simulink model "Kinematic"  (R2023b)
settings: Solver=VariableStepAuto  StartTime=0.0  StopTime=10.0  RelTol=1e-3
values from neighbouring files (symbols this model uses):
  dQ1 = x(6)    [BSM.m]    (also in Correct_new_data.m; MechanicalMechanics_Dynamic.m; MechanicalMechanics_Dynamic_adaptive_BSM.m; MechanicalMechanics_Kinematics.m)
  L1 = x(1)    [Adams_HW1.m]    (also in Adams_HW_DrawGIF.m = current_x(1); Adams_HW_DrawGIF_Y.m = current_x(1); BSM.m; Correct_new_data.m)
  L2 = x(2)    [Adams_HW1.m]    (also in Adams_HW_DrawGIF.m = current_x(2); Adams_HW_DrawGIF_Y.m = current_x(2); BSM.m; Correct_new_data.m)
  L3 = x(3)    [Adams_HW1.m]    (also in Adams_HW_DrawGIF.m = current_x(3); Adams_HW_DrawGIF_Y.m = current_x(3); BSM.m; Correct_new_data.m)
  L4 = x(4)    [Adams_HW1.m]    (also in Adams_HW_DrawGIF.m = current_x(4); Adams_HW_DrawGIF_Y.m = current_x(4); BSM.m; Correct_new_data.m)
  Q1 = x(5)    [Adams_HW1.m]    (also in Adams_HW_DrawGIF.m = current_x(5); Adams_HW_DrawGIF_Y.m = current_x(5); BSM.m; Correct_new_data.m)
  Q2 = Inition(1)    [Adams_HW1.m]    (also in BSM.m = x(8); Correct_new_data.m = x(8); GenerateSimplifiedMechanism.m = x(8); MechanicalMechanics_Dynamic.m = x(8))
  Q3 = x(11)    [Adams_HW1.m]    (also in Adams_HW_DrawGIF.m = current_x(11); Adams_HW_DrawGIF_Y.m = current_x(7); BSM.m; Correct_new_data.m)
  s = x(14)    [BSM.m]    (also in Correct_new_data.m; GenerateSimplifiedMechanism.m; MechanicalMechanics_Dynamic.m; MechanicalMechanics_Dynamic_adaptive_BSM.m)
settings Model: Creator=Akko  LastModifiedBy=Akko

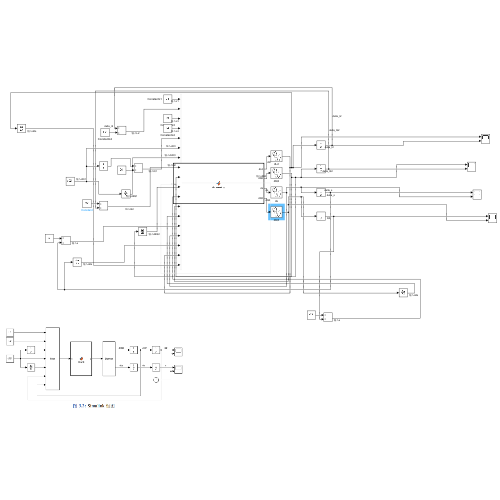
[thumbnail: Simulink's stored preview of the top-level diagram]
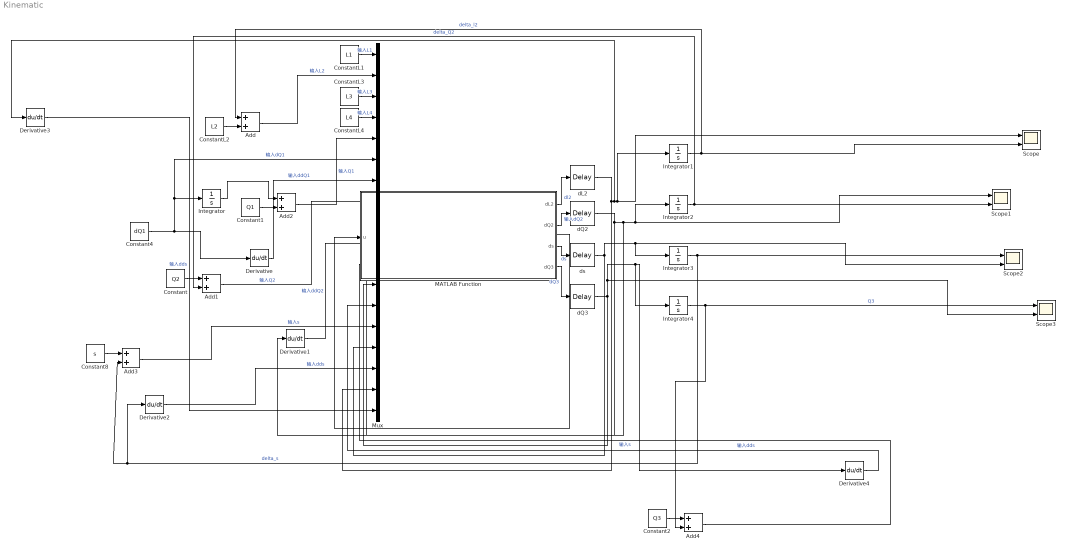
== system Kinematic ==
  Add{,1..4} (5 alike) : Sum
  Constant : Constant  Value=Q2
  Constant1 : Constant  Value=Q1
  Constant2 : Constant  Value=Q3
  Constant4 : Constant  Value=dQ1
  Constant8 : Constant  Value=s
  ConstantL1 : Constant  Value=L1
  ConstantL2 : Constant  Value=L2
  ConstantL3 : Constant  Value=L3
  ConstantL4 : Constant  Value=L4
  Derivative{,1..4} (5 alike) : Derivative
  Integrator{,1..4} (5 alike) : Integrator
  MATLAB Function : MATLAB Function  TreatAsAtomicUnit=on
  Mux : Mux  Inputs=18
  Scope{,1..3} (4 alike) : Scope  NumInputPorts=2
  dL2 : TransportDelay  DelayTime=1e-4
  dQ2 : TransportDelay  DelayTime=1e-4
  dQ3 : TransportDelay  DelayTime=1e-4
  ds : TransportDelay  DelayTime=1e-4
  wires:
  Mux/1 -> MATLAB Function/1(u)
  Integrator/1 -> Add2/1
  Constant4/1 -> Mux/6, Integrator/1, Derivative/1  "输入dQ1"
  ConstantL1/1 -> Mux/1  "输入L1"
  ConstantL2/1 -> Add/2
  ConstantL4/1 -> Mux/4  "输入L4"
  ConstantL3/1 -> Mux/3  "输入L3"
  Integrator4/1 -> Add4/2, Scope3/1  "Q3"
  Derivative/1 -> Mux/7  "输入ddQ1"
  MATLAB Function/1(dL2) -> dL2/1  "dl2"
  MATLAB Function/2(dQ2) -> dQ2/1  "输入dQ2"
  MATLAB Function/3(ds) -> ds/1  "ds"
  MATLAB Function/4(dQ3) -> dQ3/1  "dQ3"
  Integrator3/1 -> Add3/2, Derivative2/1, Scope2/1  "delta_s"
  Integrator1/1 -> Add/1, Scope/2  "delta_l2"
  Integrator2/1 -> Add1/2, Scope1/2  "delta_Q2"
  Add/1 -> Mux/2  "输入L2"
  Constant/1 -> Add1/1
  Add1/1 -> Mux/8  "输入Q2"
  Add2/1 -> Mux/5  "输入Q1"
  Constant1/1 -> Add2/2
  Derivative1/1 -> Mux/10  "输入ddQ2"
  Constant8/1 -> Add3/1
  Derivative2/1 -> Mux/16  "输入dds"
  Add3/1 -> Mux/14  "输入s"
  Constant2/1 -> Add4/1
  Add4/1 -> Mux/11  "输入s"
  Derivative4/1 -> Mux/13  "输入dds"
  Derivative3/1 -> Mux/18  "输入dds"
  dL2/1 -> Mux/17, Scope/1, Integrator1/1, Derivative3/1
  dQ2/1 -> Mux/9, Scope1/1, Integrator2/1, Derivative1/1
  ds/1 -> Scope2/2, Integrator3/1, Mux/15
  dQ3/1 -> Derivative4/1, Integrator4/1, Scope3/2, Mux/12

== matlab function Kinematic/MATLAB Function ==
  data: u input; dL2 output; dQ2 output; ds output; dQ3 output
function [dL2,dQ2,ds,dQ3]=Kinematics(u)
coder.extrinsic('MechanicalMechanics_Kinematics');
dL2 = 0; dQ2 = 0; ds = 0; dQ3 = 0;
[dL2,dQ2,ds,dQ3] = MechanicalMechanics_Kinematics(u);
end
